simulink model "SBC2"  (R2023a)
settings: Solver=VariableStepAuto  StartTime=0  StopTime=10  FixedStep=0.002  RelTol=1e-3  AbsTol=1e-6
InitFcn:
  | global t
  | t = 0;
libraries: Solver_SF x1, slpidlib x1
settings Model: ExtModeTrigMode=oneshot  Creator=ywata  LastModifiedBy=USER
settings SolverCC: AutoScaleAbsTol=off  AlgebraicLoopSolver=TrustRegion
settings DataIOCC: SaveFormat=Array  SignalLoggingSaveFormat=ModelDataLogs  ReturnWorkspaceOutputs=off  SignalLoggingName=sigsOut
settings OptimizationCC: BlockReduction=off  BooleanDataType=off  ExpressionDepthLimit=2147483647  LifeSpan=inf
settings DebuggingCC: SaveWithParameterizedLinksMsg=none  UnderspecifiedInitializationDetection=Classic  MergeDetectMultiDrivingBlocksExec=none  SignalResolutionControl=TryResolveAllWithWarning  MultiTaskDSMMsg=warning  MultiTaskCondExecSysMsg=none  FcnCallInpInsideContextMsg=warning  UnconnectedInputMsg=warning  UnconnectedOutputMsg=warning  UnconnectedLineMsg=warning  StateNameClashWarn=warning  SFUnexpectedBacktrackingDiag=warning  SFNoUnconditionalDefaultTransitionDiag=warning  SFExecutionAtInitializationDiag=none  ArithmeticOperatorsInVariantConditions=warning
settings HardwareCC: ProdBitPerPointer=32  ProdBitPerSizeT=32  ProdBitPerPtrDiffT=32  ProdLargestAtomicFloat=None  ProdIntDivRoundTo=Undefined  ProdEndianess=Unspecified  ProdWordSize=32  ProdHWDeviceType=32-bit Generic  TargetUnknown=on
settings ModelReferenceCC: PropagateSignalLabelsOutOfModel=off
settings SFSimCC: SimUseLocalCustomCode=off  CustomCodeUndefinedFunction=UseInterfaceOnly
settings RTWCC: TemplateMakefile=grt_vc.tmf  RTWUseLocalCustomCode=off
settings CodeAppCC: StateflowObjectComments=on
settings GRTTargetCC: TargetFcnLib=ansi_tfl_tmw.mat  TargetLangStandard=C89/C90 (ANSI)  CombineOutputUpdateFcns=off  GRTInterface=on
settings ConfigComp: CovMetricSettings=dw  CovSaveCumulativeToWorkspaceVar=on  CovSaveSingleToWorkspaceVar=on  CovExternalEMLEnable=off

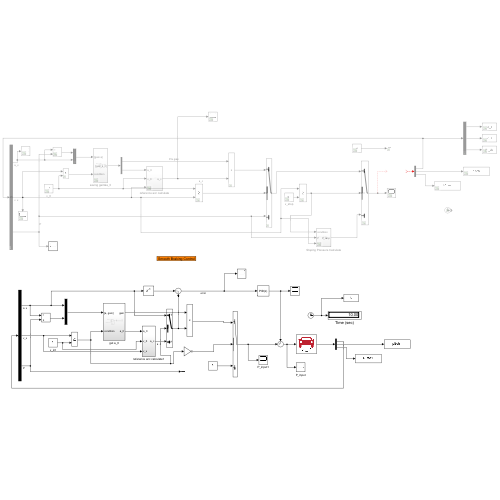
[thumbnail: Simulink's stored preview of the top-level diagram]
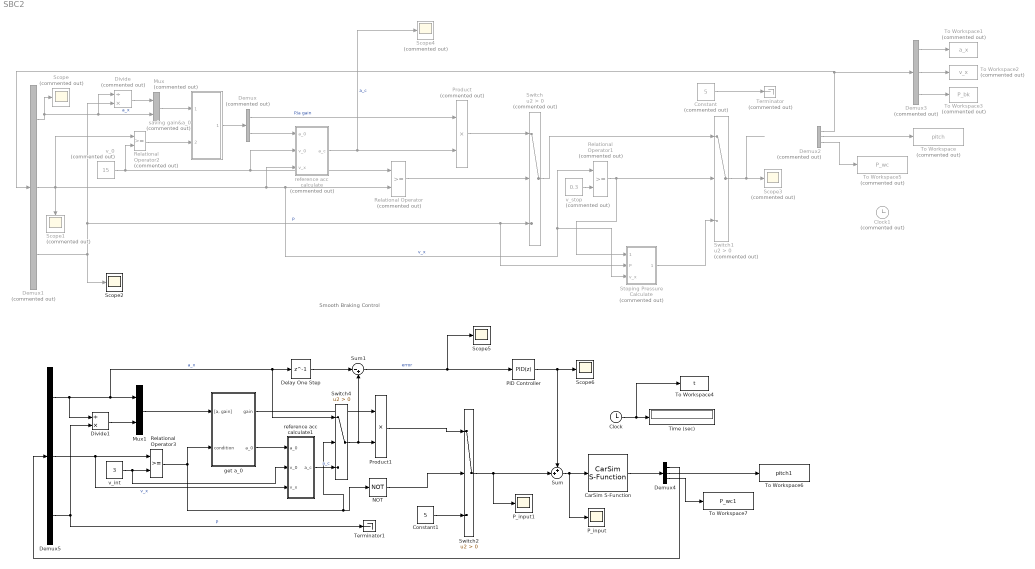
== system SBC2 ==
  note: Smooth Braking Control
  CarSim S-Function : Solver_SF/CarSim S-Function  Priority=1  SIMFILE=simfile.sim  Run_RTs=off  vs_state_ind=Run  StopMode_ind=Vehicle Model
  Clock : Clock
  Clock1 : Clock  Commented=on
  Constant : Constant  Commented=on  Value=5
  Constant1 : Constant  Value=5
  Delay One Step : Delay  DelayLength=1
  Demux : Demux  Commented=on  Outputs=2
  Demux1 : Demux  Commented=on  Outputs=3
      settings: DisplayOption=none
  Demux2 : Demux  Commented=on  Outputs=[3 1 4]
  Demux3 : Demux  Commented=on  Outputs=3
  Demux4 : Demux  Outputs=[3 1 4]
  Demux5 : Demux  Outputs=3
      settings: DisplayOption=none
  Divide : Product  Commented=on  Inputs=/*
  Divide1 : Product  Inputs=/*
  Mux : Mux  Commented=on  Inputs=2
  Mux1 : Mux  Inputs=2
  NOT : Logic  Operator=NOT  IconShape=distinctive  AllPortsSameDT=off  OutDataTypeStr=boolean
  PID Controller : slpidlib/PID Controller  Controller=PID  Form=Parallel  TimeDomain=Discrete-time  UseExternalTs=off  SampleTime=-1  IntegratorMethod=Forward Euler  FilterMethod=Forward Euler  ControllerParametersSource=internal  P=0.01  I=0.05  UseKiTs=on  D=0  N=100  UseFilter=on  TunerSelectOption=Transfer Function Based (PID Tuner App)  InitialConditionSource=internal  InitialConditionForIntegrator=0  InitialConditionForFilter=0  DifferentiatorICPrevScaledInput=0  ExternalReset=none  TrackingMode=off  Kt=1  LimitOutput=off  SatLimitsSource=internal  UpperSaturationLimit=inf  LowerSaturationLimit=-inf  LinearizeAsGain=on  AntiWindupMode=none  Kb=1  LimitIntegrator=off  UpperIntegratorSaturationLimit=inf  LowerIntegratorSaturationLimit=-inf  POutMin=[]  POutMax=[]  IOutMin=[]  IOutMax=[]  DOutMin=[]  DOutMax=[]  NOutMin=[]  NOutMax=[]  SumOutMin=[]  SumOutMax=[]  SaturationOutMin=[]  SaturationOutMax=[]  PParamMin=[]  PParamMax=[]  IParamMin=[]  IParamMax=[]  DParamMin=[]  DParamMax=[]  NParamMin=[]  NParamMax=[]  KbParamMin=[]  KbParamMax=[]  KtParamMin=[]  KtParamMax=[]  KbOutMin=[]  KbOutMax=[]  KtOutMin=[]  KtOutMax=[]  IntegratorOutMin=[]  IntegratorOutMax=[]  FilterOutMin=[]  FilterOutMax=[]  SumI1OutMin=[]  SumI1OutMax=[]  SumI2OutMin=[]  SumI2OutMax=[]  SumI3OutMin=[]  SumI3OutMax=[]  SumI4OutMin=[]  SumI4OutMax=[]  SumDOutMin=[]  SumDOutMax=[]  DifferentiatorOutMin=[]  DifferentiatorOutMax=[]  FilterDiffOutCoefMin=[]  FilterDiffOutCoefMax=[]  ReciprocalOutMin=[]  ReciprocalOutMax=[]  SumDenOutMin=[]  SumDenOutMax=[]  SumNumOutMin=[]  SumNumOutMax=[]  DivideOutMin=[]  DivideOutMax=[]  UdiffTsProdOutMin=[]  UdiffTsProdOutMax=[]  NTsProdOutMin=[]  NTsProdOutMax=[]  UintegralTsProdOutMin=[]  UintegralTsProdOutMax=[]  UngainTsProdOutMin=[]  UngainTsProdOutMax=[]  ClampingZeroOutDataTypeStr=Inherit: Inherit via back propagation  ClampingZeroOutMin=[]  ClampingZeroOutMax=[]  FilterDenConstantOutDataTypeStr=Inherit: Inherit via back propagation  FilterDenConstantOutMin=[]  FilterDenConstantOutMax=[]  PCopyOutDataTypeStr=Inherit: Inherit via back propagation  PCopyOutMin=[]  PCopyOutMax=[]  NCopyOutDataTypeStr=Inherit: Inherit via back propagation  NCopyOutMin=[]  NCopyOutMax=[]  IntegratorContinuousStateAttributes=''  IntegratorStateMustResolveToSignalObject=off  IntegratorRTWStateStorageClass=Auto  FilterContinuousStateAttributes=''  FilterStateMustResolveToSignalObject=off  FilterRTWStateStorageClass=Auto  ParallelPVariant=InternalParameters  IdealPVariant=Disabled  IVariant=InternalParameters  DVariant=InternalParameters  IntegratorVariant=Discrete  SatVariant=Disabled  AWVariant=Passthrough  PCopyVariant=Disabled  TRVariant=Disabled  FdbkBlocksVariant=Forward  IdealPFdbkVariant=Disabled  SatFdbkVariant=Disabled  DerivativeFilterVariant=ForwardEulerFilter  NVariant=InternalParameters  NCopyVariant=Disabled  FilterICVariant=InternalICsFilter  IntegratorICVariant=InternalICs  ExternalResetVariant=Disabled  TRSumVariant=Passthrough  SumFdbkVariant=Disabled  SumVariant=Sum_PID  TsampFilterVariant=InternalTs  TsampNgainVariant=Passthrough  TsampIntegralVariant=Disabled_SignalSpec  ExternalSaturationOutDataTypeStr=Inherit: Same as second input
  P_input : Scope
  P_input1 : Scope
  Product : Product  Commented=on
  Product1 : Product
  Relational Operator : RelationalOperator  Commented=on  OutDataTypeStr=boolean  RndMeth=Simplest  InputSameDT=off
  Relational Operator1 : RelationalOperator  Commented=on  OutDataTypeStr=boolean  RndMeth=Simplest  InputSameDT=off
  Relational Operator2 : RelationalOperator  Commented=on  OutDataTypeStr=boolean  RndMeth=Simplest  InputSameDT=off
  Relational Operator3 : RelationalOperator  OutDataTypeStr=boolean  RndMeth=Simplest  InputSameDT=off
  Scope{,1,3..4} (4 alike) : Scope  Commented=on
  Scope2 : Scope
  Scope5 : Scope
  Scope6 : Scope
  Stoping Pressure Calculate : Subsystem  Commented=on
  Sum : Sum  Inputs=++|
  Sum1 : Sum  Inputs=|-+
  Switch : Switch  Commented=on  Criteria=u2 > Threshold  SaturateOnIntegerOverflow=off  InputSameDT=off
  Switch1 : Switch  Commented=on  Criteria=u2 > Threshold  SaturateOnIntegerOverflow=off  InputSameDT=off
  Switch2 : Switch  Criteria=u2 > Threshold  SaturateOnIntegerOverflow=off  InputSameDT=off
  Switch4 : Switch  Criteria=u2 > Threshold  SaturateOnIntegerOverflow=off  InputSameDT=off
  Terminator : Terminator  Commented=on
  Terminator1 : Terminator
  Time (sec) : Display
      settings: Format=bank  Decimation=100
  To Workspace : ToWorkspace  Commented=on  VariableName=pitch  SaveFormat=Timeseries  SampleTime=-1
  To Workspace1 : ToWorkspace  Commented=on  VariableName=a_x  SaveFormat=Timeseries  SampleTime=-1
  To Workspace2 : ToWorkspace  Commented=on  VariableName=v_x  SaveFormat=Timeseries  SampleTime=-1
  To Workspace3 : ToWorkspace  Commented=on  VariableName=P_bk  SaveFormat=Timeseries  SampleTime=-1
  To Workspace4 : ToWorkspace  VariableName=t  SaveFormat=Timeseries  SampleTime=-1
  To Workspace5 : ToWorkspace  Commented=on  VariableName=P_wc  SaveFormat=Timeseries  SampleTime=-1
  To Workspace6 : ToWorkspace  VariableName=pitch1  SaveFormat=Timeseries  SampleTime=-1
  To Workspace7 : ToWorkspace  VariableName=P_wc1  SaveFormat=Timeseries  SampleTime=-1
  get a_0 : Subsystem
  reference acc calculate : Subsystem  Commented=on
  reference acc calculate1 : Subsystem
  saving gain&a_0 : Subsystem  Commented=on
  v_0 : Constant  Commented=on  Value=15
  v_int : Constant  Value=3
  v_stop : Constant  Commented=on  Value=0.3
  wires:
  Clock/1 -> To Workspace4/1, Time (sec)/1
  Demux1/3 -> Scope2/1, Divide/2, Stoping Pressure Calculate/2(P), Switch/3  "P"
  Demux1/1 -> Scope/1, Divide/1, Mux/2  "a_x"
  Demux1/2 -> reference acc calculate/3(v_x), Stoping Pressure Calculate/3(v_x), Relational Operator1/1, Relational Operator/2, Scope1/1, Relational Operator2/1  "v_x"
  v_0/1 -> Relational Operator2/2, reference acc calculate/2(v_0), Relational Operator/1
  reference acc calculate/1(a_c) -> Scope4/1, Product/2  "a_c"
  Relational Operator/1 -> Switch/2
  Switch/1 -> Switch1/1
  Relational Operator1/1 -> Stoping Pressure Calculate/1(condition), Switch1/2
  v_stop/1 -> Relational Operator1/2
  Divide/1 -> Mux/1
  Demux/2 -> reference acc calculate/1(a_0)
  Product/1 -> Switch/1
  Demux/1 -> Product/1  "P/a gain"
  Switch1/1 -> Scope3/1
  Demux2/1 -> Demux1/1, Demux3/1
  Stoping Pressure Calculate/1(P_stop) -> Switch1/3
  Mux/1 -> saving gain&a_0/1("[gain a]")
  Relational Operator2/1 -> saving gain&a_0/2(condition)
  saving gain&a_0/1("[gain a_0]") -> Demux/1
  ? -> Demux2/1
  Demux2/2 -> To Workspace/1
  Demux3/1 -> To Workspace1/1
  Demux3/2 -> To Workspace2/1
  Demux3/3 -> To Workspace3/1
  Constant/1 -> Terminator/1
  Demux2/3 -> To Workspace5/1
  Demux4/3 -> To Workspace7/1
  Demux4/2 -> To Workspace6/1
  CarSim S-Function/1 -> Demux4/1
  Demux4/1 -> Demux5/1
  Demux5/2 -> reference acc calculate1/3(v_x), Relational Operator3/1  "v_x"
  v_int/1 -> reference acc calculate1/2(v_0), Relational Operator3/2
  Demux5/1 -> Divide1/1, Switch4/1, Delay One Step/1, Mux1/1  "a_x"
  Relational Operator3/1 -> get a_0/2(condition), NOT/1, Switch4/2
  Demux5/3 -> Terminator1/1, Divide1/2  "P"
  Divide1/1 -> Mux1/2
  Mux1/1 -> get a_0/1("[a, gain]")
  get a_0/2(a_0) -> reference acc calculate1/1(a_0)
  get a_0/1(gain) -> Product1/1
  Product1/1 -> Switch2/1
  NOT/1 -> Switch2/2
  Switch2/1 -> P_input1/1, Sum/2
  Delay One Step/1 -> Sum1/1
  Sum1/1 -> Scope5/1, PID Controller/1  "error"
  Sum/1 -> P_input/1, CarSim S-Function/1
  PID Controller/1 -> Sum/1, Scope6/1
  reference acc calculate1/1(a_c) -> Switch4/3  "a_c"
  Switch4/1 -> Sum1/2, Product1/2
  Constant1/1 -> Switch2/3

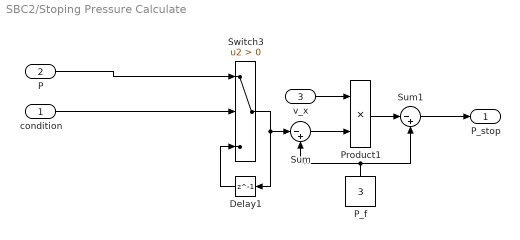
== system SBC2/Stoping Pressure Calculate ==
  condition : Inport
  P : Inport  Port=2
  v_x : Inport  Port=3
  Delay1 : Delay  DelayLength=1  InitialCondition=0
  P_f : Constant  Value=3
  Product1 : Product
  Sum : Sum  Inputs=|-+
  Sum1 : Sum  Inputs=|-+
  Switch3 : Switch  Criteria=u2 > Threshold  SaturateOnIntegerOverflow=off  InputSameDT=off
  P_stop : Outport
  wires:
  Product1/1 -> Sum1/1
  Switch3/1 -> Sum/1, Delay1/1
  Delay1/1 -> Switch3/3
  condition/1 -> Switch3/2
  P_f/1 -> Sum/2, Sum1/2
  Sum1/1 -> P_stop/1
  Sum/1 -> Product1/2
  P/1 -> Switch3/1
  v_x/1 -> Product1/1

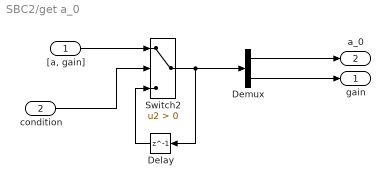
== system SBC2/get a_0 ==
  "[a, gain]" : Inport
  condition : Inport  Port=2
  Delay : Delay  DelayLength=1  InitialCondition=0
  Demux : Demux  Outputs=2
  Switch2 : Switch  Criteria=u2 > Threshold  SaturateOnIntegerOverflow=off  InputSameDT=off
  gain : Outport
  a_0 : Outport  Port=2
  wires:
  Switch2/1 -> Demux/1, Delay/1
  Delay/1 -> Switch2/3
  condition/1 -> Switch2/2
  "[a, gain]"/1 -> Switch2/1
  Demux/2 -> gain/1
  Demux/1 -> a_0/1

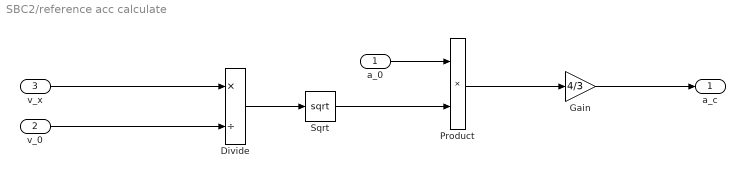
== system SBC2/reference acc calculate ==
  a_0 : Inport
  v_0 : Inport  Port=2
  v_x : Inport  Port=3
  Divide : Product  Inputs=*/
  Gain : Gain  Gain=4/3
  Product : Product
  Sqrt : Sqrt
  a_c : Outport
  wires:
  v_x/1 -> Divide/1
  v_0/1 -> Divide/2
  Divide/1 -> Sqrt/1
  Sqrt/1 -> Product/2
  a_0/1 -> Product/1
  Product/1 -> Gain/1
  Gain/1 -> a_c/1

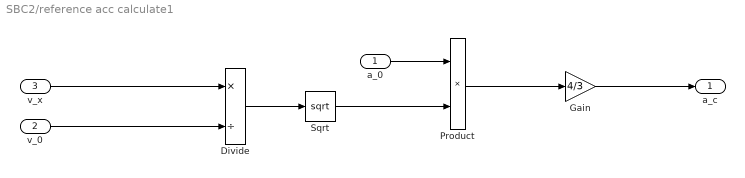
== system SBC2/reference acc calculate1 ==
  a_0 : Inport
  v_0 : Inport  Port=2
  v_x : Inport  Port=3
  Divide : Product  Inputs=*/
  Gain : Gain  Gain=4/3
  Product : Product
  Sqrt : Sqrt
  a_c : Outport
  wires:
  v_x/1 -> Divide/1
  v_0/1 -> Divide/2
  Divide/1 -> Sqrt/1
  Sqrt/1 -> Product/2
  a_0/1 -> Product/1
  Product/1 -> Gain/1
  Gain/1 -> a_c/1

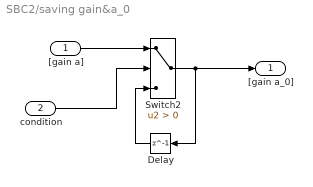
== system SBC2/saving gain&a_0 ==
  "[gain a]" : Inport
  condition : Inport  Port=2
  Delay : Delay  DelayLength=1  InitialCondition=0
  Switch2 : Switch  Criteria=u2 > Threshold  SaturateOnIntegerOverflow=off  InputSameDT=off
  "[gain a_0]" : Outport
  wires:
  Switch2/1 -> "[gain a_0]"/1, Delay/1
  Delay/1 -> Switch2/3
  condition/1 -> Switch2/2
  "[gain a]"/1 -> Switch2/1
